simulink model "nlin_2DoF1"  (R2025a)
settings: Solver=VariableStepAuto  StartTime=0.0  StopTime=100  RelTol=1e-3
settings Model: Creator=ASUS  LastModifiedBy=jidki

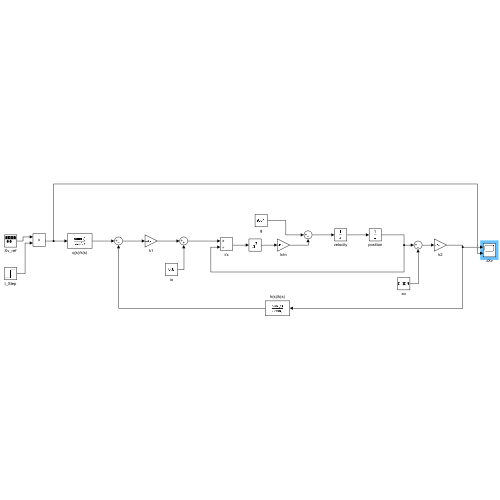
[thumbnail: Simulink's stored preview of the top-level diagram]
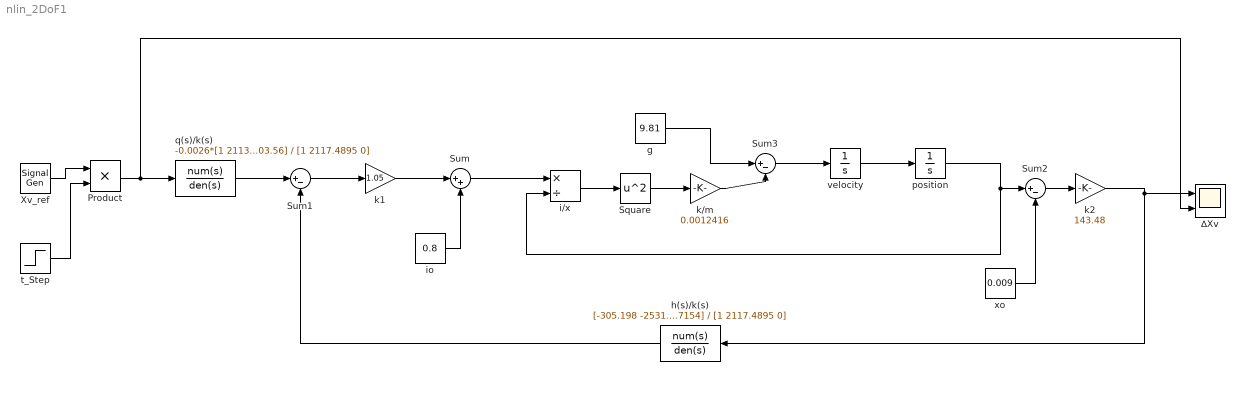
== system nlin_2DoF1 ==
  Product : Product
  Square : Math  Operator=square
  Sum : Sum  Inputs=|++
  Sum1 : Sum  Inputs=|+-
  Sum2 : Sum  Inputs=|+-
  Sum3 : Sum  Inputs=|+-
  Xv_ref : SignalGenerator  WaveForm=square  Frequency=1/5  Units=rad/sec
  g : Constant  Value=9.81
  h(s)/k(s) : TransferFcn  Numerator=[-305.198 -2531.996 -2834.57154]  Denominator=[1 2117.4895 0]
  i/x : Product  Inputs=*/
  io : Constant  Value=0.8
  k/m : Gain  Gain=0.0012416
  k1 : Gain  Gain=1.05
  k2 : Gain  Gain=143.48
  position : Integrator  InitialCondition=0.009
  q(s)/k(s) : TransferFcn  Numerator=-0.0026*[1 2113.2 1116403.56]  Denominator=[1 2117.4895 0]
  t_Step : Step  Time=25  SampleTime=0
  velocity : Integrator
  xo : Constant  Value=0.009
  ∆Xv : Scope  NumInputPorts=2
      settings: ActiveDisplayYMinimum=-1.4107099360273823  ActiveDisplayYMaximum=1.4096466731911588
  wires:
  io/1 -> Sum/2
  i/x/1 -> Square/1
  Square/1 -> k/m/1
  k/m/1 -> Sum3/2
  velocity/1 -> position/1
  position/1 -> Sum2/1, i/x/2
  xo/1 -> Sum2/2
  Sum2/1 -> k2/1
  k2/1 -> h(s)/k(s)/1, ∆Xv/1
  Sum1/1 -> k1/1
  h(s)/k(s)/1 -> Sum1/2
  q(s)/k(s)/1 -> Sum1/1
  Product/1 -> ∆Xv/2, q(s)/k(s)/1
  Xv_ref/1 -> Product/1
  t_Step/1 -> Product/2
  Sum/1 -> i/x/1
  g/1 -> Sum3/1
  Sum3/1 -> velocity/1
  k1/1 -> Sum/1
